simulink model "onhangolo_szabalyzok"  (R2018a)
settings: Solver=VariableStepAuto  StartTime=0.0  StopTime=500  RelTol=1e-3
libraries: simulink x2
settings Model: Creator=alfac  LastModifiedBy=hamar

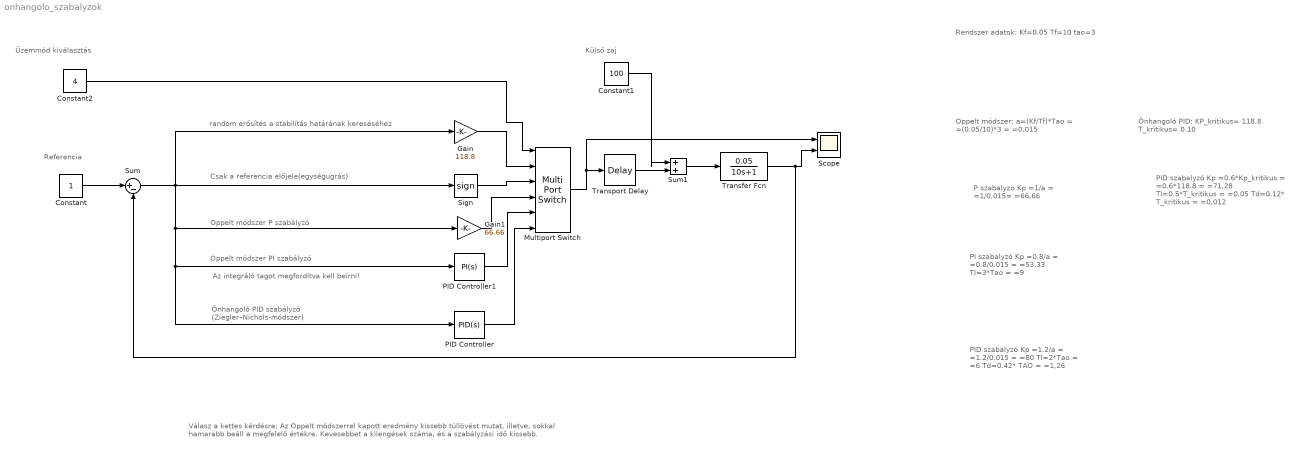
== system onhangolo_szabalyzok ==
  note: Az integráló tagot megfordítva kell beírni!
  note: Oppelt módszer PI szabályzó
  note: PID szabalyzó
      | Kp =1.2/a =
      | =1.2/0.015 =
      | =80
      | TI=2*Tao =
      | =6
      | Td=0.42* TAO =
      | =1,26
  note: Rendszer adatok:
      | Kf=0.05
      | Tf=10
      | tao=3
  note: Oppelt módszer:
      | a=(Kf/Tf)*Tao =
      | =(0.05/10)*3 =
      | =0,015
  note: P szabalyzo
      | Kp =1/a =
      | =1/0.015=
      | =66,66
  note: PI szabalyzó
      | Kp =0.8/a =
      | =0.8/0.015 =
      | =53,33
      | TI=3*Tao =
      | =9
  note: Oppelt módszer P szabályzó
  note: Üzemmód kiválasztás
  note: random erősítés a stabilítás
      | határának kereséséhez
  note: Csak a referencia előjele(egységugrás)
  note: Önhangoló PID:
      | KP_kritikus= 118.8
      | T_kritikus= 0.10
  note: PID szabalyzó
      | Kp =0.6*Kp_kritikus =
      | =0.6*118.8 =
      | =71,28
      | TI=0.5*T_kritikus =
      | =0,05
      | Td=0.12* T_kritikus =
      | =0,012
  note: Önhangoló PID szabályzó
      | (Ziegler–Nichols-módszer)
  note: Referencia
  note: Külső zaj
  note: Válasz a kettes kérdésre: Az Oppelt módszerrel kapott eredmény kissebb túllövést mutat, illetve, sokkal
      | hamarabb beáll a megfelelő értékre. Kevesebbet a kilengések száma, és a szabályzási idő kissebb.
  Constant : Constant
  Constant1 : Constant  Value=100
  Constant2 : Constant  Value=4
  Gain : Gain  Gain=118.8
  Gain1 : Gain  Gain=66.66
  Multiport Switch : MultiPortSwitch  Inputs=5
  PID Controller : simulink/Continuous/PID Controller  Controller=PID  TimeDomain=Continuous-time  SampleTime=-1  IntegratorMethod=Forward Euler  FilterMethod=Forward Euler  Form=Ideal  UseFilter=on  ControllerParametersSource=internal  P=71.28  I=0.05  D=0.012  N=100  InitialConditionSource=internal  InitialConditionForIntegrator=0  InitialConditionForFilter=0  ExternalReset=none  LimitOutput=off  UpperSaturationLimit=inf  LowerSaturationLimit=-inf  LinearizeAsGain=on  AntiWindupMode=none  Kb=1  TrackingMode=off  Kt=1  PParamMin=[]  PParamMax=[]  IParamMin=[]  IParamMax=[]  DParamMin=[]  DParamMax=[]  NParamMin=[]  NParamMax=[]  KbParamMin=[]  KbParamMax=[]  KtParamMin=[]  KtParamMax=[]  POutMin=[]  POutMax=[]  IOutMin=[]  IOutMax=[]  DOutMin=[]  DOutMax=[]  NOutMin=[]  NOutMax=[]  KbOutMin=[]  KbOutMax=[]  KtOutMin=[]  KtOutMax=[]  IntegratorOutMin=[]  IntegratorOutMax=[]  FilterOutMin=[]  FilterOutMax=[]  SumOutMin=[]  SumOutMax=[]  SumI1OutMin=[]  SumI1OutMax=[]  SumI2OutMin=[]  SumI2OutMax=[]  SumI3OutMin=[]  SumI3OutMax=[]  SumDOutMin=[]  SumDOutMax=[]  SaturationOutMin=[]  SaturationOutMax=[]  IntegratorContinuousStateAttributes=''  IntegratorStateMustResolveToSignalObject=off  IntegratorRTWStateStorageClass=Auto  FilterContinuousStateAttributes=''  FilterStateMustResolveToSignalObject=off  FilterRTWStateStorageClass=Auto  DifferentiatorICPrevScaledInput=0  DifferentiatorOutMin=[]  DifferentiatorOutMax=[]  FilterDiffOutCoefMin=[]  FilterDiffOutCoefMax=[]  SumDenOutMin=[]  SumDenOutMax=[]  SumNumOutMin=[]  SumNumOutMax=[]  ReciprocalOutMin=[]  ReciprocalOutMax=[]  DivideOutMin=[]  DivideOutMax=[]  TunerSelectOption=Transfer Function Based (PID Tuner App)
  PID Controller1 : simulink/Continuous/PID Controller  Controller=PI  TimeDomain=Continuous-time  SampleTime=-1  IntegratorMethod=Forward Euler  FilterMethod=Forward Euler  Form=Ideal  UseFilter=on  ControllerParametersSource=internal  P=53.33  I=1/9  D=1  N=100  InitialConditionSource=internal  InitialConditionForIntegrator=0  InitialConditionForFilter=0  ExternalReset=none  LimitOutput=off  UpperSaturationLimit=inf  LowerSaturationLimit=-inf  LinearizeAsGain=on  AntiWindupMode=none  Kb=1  TrackingMode=off  Kt=1  PParamMin=[]  PParamMax=[]  IParamMin=[]  IParamMax=[]  DParamMin=[]  DParamMax=[]  NParamMin=[]  NParamMax=[]  KbParamMin=[]  KbParamMax=[]  KtParamMin=[]  KtParamMax=[]  POutMin=[]  POutMax=[]  IOutMin=[]  IOutMax=[]  DOutMin=[]  DOutMax=[]  NOutMin=[]  NOutMax=[]  KbOutMin=[]  KbOutMax=[]  KtOutMin=[]  KtOutMax=[]  IntegratorOutMin=[]  IntegratorOutMax=[]  FilterOutMin=[]  FilterOutMax=[]  SumOutMin=[]  SumOutMax=[]  SumI1OutMin=[]  SumI1OutMax=[]  SumI2OutMin=[]  SumI2OutMax=[]  SumI3OutMin=[]  SumI3OutMax=[]  SumDOutMin=[]  SumDOutMax=[]  SaturationOutMin=[]  SaturationOutMax=[]  IntegratorContinuousStateAttributes=''  IntegratorStateMustResolveToSignalObject=off  IntegratorRTWStateStorageClass=Auto  FilterContinuousStateAttributes=''  FilterStateMustResolveToSignalObject=off  FilterRTWStateStorageClass=Auto  DifferentiatorICPrevScaledInput=0  DifferentiatorOutMin=[]  DifferentiatorOutMax=[]  FilterDiffOutCoefMin=[]  FilterDiffOutCoefMax=[]  SumDenOutMin=[]  SumDenOutMax=[]  SumNumOutMin=[]  SumNumOutMax=[]  ReciprocalOutMin=[]  ReciprocalOutMax=[]  DivideOutMin=[]  DivideOutMax=[]  TunerSelectOption=Transfer Function Based (PID Tuner App)
  Scope : Scope  NumInputPorts=2
  Sign : Signum
  Sum : Sum  Inputs=|+-
  Sum1 : Sum  Inputs=|++
  Transfer Fcn : TransferFcn  Numerator=[0.05]  Denominator=[10 1]
  Transport Delay : TransportDelay  DelayTime=3
  wires:
  Constant/1 -> Sum/1
  Sum/1 -> Sign/1, PID Controller/1, PID Controller1/1, Gain1/1, Gain/1
  Constant2/1 -> Multiport Switch/1
  Gain/1 -> Multiport Switch/2
  Sign/1 -> Multiport Switch/3
  Multiport Switch/1 -> Scope/1, Transport Delay/1
  Transfer Fcn/1 -> Scope/2, Sum/2
  Gain1/1 -> Multiport Switch/4
  PID Controller1/1 -> Multiport Switch/5
  PID Controller/1 -> Multiport Switch/6
  Constant1/1 -> Sum1/1
  Transport Delay/1 -> Sum1/2
  Sum1/1 -> Transfer Fcn/1
